simulink model "sampleModel2072_pp_difftest"  (R2021a)
settings: Solver=VariableStepAuto  StartTime=0.0  StopTime=10.0  RelTol=1e-3
undefined symbols (not defined in the file or in its folder): DiscIntNeverNeededParam, magnitude, Newton, Raphson
libraries: simulink x184, pid_lib x33
(part 5 of 5)

== system sampleModel2072_pp_difftest/cfblk57/cfblk10 ==
  cfblk1 : Inport
  cfblk10 : Delay  SampleTime=1
  cfblk11 : Delay  SampleTime=1
  cfblk3 : Delay  ShowEnablePort=on  SampleTime=1
      settings: InputPortMap=u0,e6
  cfblk4 : simulink/Discrete/Difference  ICPrevInput=0.0  OutMin=[]  OutMax=[]  OutDataTypeStr=Inherit: Inherit via back propagation  OutDataType=fixdt(1, 16)  OutScaling=2^-10  DoSatur=off
  cfblk5 : simulink/Discrete/Transfer Fcn Lead or Lag  PoleZ=0.95  ZeroZ=0.75  ICPrevOutput=0.0  ICPrevInput=0.0  DoSatur=off
      settings: SourceProductBaseCode=SL
  cfblk6 : Sqrt  SaturateOnIntegerOverflow=on
  cfblk7 : Product
  cfblk8 : Sum  Inputs=+-
  cfblk9 : Polyval  Coefs=[ +2.081618890e-019, -1.441693666e-014, +4.719686976e-010, -8.536869453e-006, +1.621573104e-001, -8.087801117e+001 ]
  cfblk2 : Outport
  wires:
  cfblk9/1 -> cfblk7/1
  cfblk1/1 -> cfblk4/1
  cfblk5/1 -> cfblk9/1
  cfblk8/1 -> cfblk6/1
  cfblk4/1 -> cfblk3/1, cfblk8/2, cfblk2/1
  cfblk3/1 -> cfblk7/2, cfblk5/1
  cfblk7/1 -> cfblk10/1
  cfblk10/1 -> cfblk3/2
  cfblk6/1 -> cfblk11/1
  cfblk11/1 -> cfblk8/1

== system sampleModel2072_pp_difftest/cfblk57/cfblk11 ==
  cfblk1 : Inport
  cfblk10 : ComplexToRealImag
  cfblk11 : Product
  cfblk12 : simulink/Math Operations/Slider Gain  gain=1  low=0  high=2
  cfblk13 : Squeeze
  cfblk14 : Product  Inputs=*
  cfblk15 : simulink/Math Operations/Slider Gain  gain=1  low=0  high=2
  cfblk16 : Delay  SampleTime=1
  cfblk3 : simulink/Discrete/Difference  ICPrevInput=0.0  OutMin=[]  OutMax=[]  OutDataTypeStr=Inherit: Inherit via back propagation  OutDataType=fixdt(1, 16)  OutScaling=2^-10  DoSatur=off
  cfblk4 : Delay  SampleTime=1
  cfblk5 : pid_lib/PID Controller (2DOF)  Controller=PID  Form=Parallel  TimeDomain=Discrete-time  UseExternalTs=off  SampleTime=1  IntegratorMethod=Forward Euler  FilterMethod=Forward Euler  ControllerParametersSource=internal  P=1  I=1  D=0  UseFilter=on  N=100  b=1  c=1  TunerSelectOption=Transfer Function Based (PID Tuner App)  InitialConditionSource=internal  InitialConditionForIntegrator=0  InitialConditionForFilter=0  DifferentiatorICPrevScaledInput=0  ExternalReset=none  TrackingMode=off  Kt=1  LimitOutput=off  SatLimitsSource=internal  UpperSaturationLimit=inf  LowerSaturationLimit=-inf  LinearizeAsGain=off  AntiWindupMode=none  Kb=1  POutMin=[]  POutMax=[]  IOutMin=[]  IOutMax=[]  DOutMin=[]  DOutMax=[]  NOutMin=[]  NOutMax=[]  bOutMin=[]  bOutMax=[]  cOutMin=[]  cOutMax=[]  SumOutMin=[]  SumOutMax=[]  SaturationOutMin=[]  SaturationOutMax=[]  PParamMin=[]  PParamMax=[]  IParamMin=[]  IParamMax=[]  DParamMin=[]  DParamMax=[]  NParamMin=[]  NParamMax=[]  bParamMin=[]  bParamMax=[]  cParamMin=[]  cParamMax=[]  KbParamMin=[]  KbParamMax=[]  KtParamMin=[]  KtParamMax=[]  KbOutMin=[]  KbOutMax=[]  KtOutMin=[]  KtOutMax=[]  IntegratorOutMin=[]  IntegratorOutMax=[]  FilterOutMin=[]  FilterOutMax=[]  SumI1OutMin=[]  SumI1OutMax=[]  SumI2OutMin=[]  SumI2OutMax=[]  SumI3OutMin=[]  SumI3OutMax=[]  SumI4OutMin=[]  SumI4OutMax=[]  SumDOutMin=[]  SumDOutMax=[]  Sum1OutMin=[]  Sum1OutMax=[]  Sum2OutMin=[]  Sum2OutMax=[]  Sum3OutMin=[]  Sum3OutMax=[]  DifferentiatorOutMin=[]  DifferentiatorOutMax=[]  FilterDiffOutCoefMin=[]  FilterDiffOutCoefMax=[]  ReciprocalOutMin=[]  ReciprocalOutMax=[]  SumDenOutMin=[]  SumDenOutMax=[]  SumNumOutMin=[]  SumNumOutMax=[]  DivideOutMin=[]  DivideOutMax=[]  UdiffTsProdOutMin=[]  UdiffTsProdOutMax=[]  NTsProdOutMin=[]  NTsProdOutMax=[]  UintegralTsProdOutMin=[]  UintegralTsProdOutMax=[]  UngainTsProdOutMin=[]  UngainTsProdOutMax=[]  IntegratorContinuousStateAttributes=''  IntegratorStateMustResolveToSignalObject=off  IntegratorRTWStateStorageClass=Auto  FilterContinuousStateAttributes=''  FilterStateMustResolveToSignalObject=off  FilterRTWStateStorageClass=Auto  ParallelPVariant=InternalParameters  IdealPVariant=Disabled  IVariant=InternalParameters  DVariant=InternalParameters  bVariant=InternalParameters  cVariant=InternalParameters  IntegratorVariant=Discrete  SatVariant=Disabled  AWVariant=Passthrough  PCopyVariant=Disabled  TRVariant=Disabled  FdbkBlocksVariant=Forward  IdealPFdbkVariant=Disabled  SatFdbkVariant=Disabled  DerivativeFilterVariant=ForwardEulerFilter  NVariant=InternalParameters  NCopyVariant=Disabled  FilterICVariant=InternalICsFilter  IntegratorICVariant=InternalICs  ExternalResetVariant=Disabled  TRSumVariant=Passthrough  SumFdbkVariant=Disabled  SumVariant=Sum_PID  TsampFilterVariant=InternalTs  TsampNgainVariant=Passthrough  TsampIntegralVariant=Passthrough  ExternalSaturationOutDataTypeStr=Inherit: Same as second input
      settings: SourceProductBaseCode=SL
  cfblk6 : Sqrt  SaturateOnIntegerOverflow=on
  cfblk7 : PermuteDimensions
  cfblk8 : Sqrt  SaturateOnIntegerOverflow=on
  cfblk9 : Math  Operator=log10  SaturateOnIntegerOverflow=on
  cfblk2 : Outport
  wires:
  cfblk11/1 -> cfblk10/1
  cfblk1/1 -> cfblk14/1
  cfblk3/1 -> cfblk5/1
  cfblk15/1 -> cfblk4/1
  cfblk7/1 -> cfblk8/1, cfblk11/2
  cfblk5/1 -> cfblk2/1
  cfblk12/1 -> cfblk13/1
  cfblk14/1 -> cfblk7/1
  cfblk4/1 -> cfblk9/1
  cfblk10/1 -> cfblk15/1
  cfblk13/1 -> cfblk5/2
  cfblk9/1 -> cfblk12/1
  cfblk6/1 -> cfblk3/1
  cfblk8/1 -> cfblk6/1
  cfblk10/2 -> cfblk16/1
  cfblk16/1 -> cfblk11/1

== system sampleModel2072_pp_difftest/cfblk57/cfblk12 ==
  cfblk1 : Inport
  cfblk10 : simulink/Math Operations/MinMax Running Resettable  Function=min  vinit=0.0
  cfblk11 : Sum  Inputs=+-
  cfblk12 : simulink/Math Operations/Slider Gain  gain=1  low=0  high=2
  cfblk13 : Squeeze
  cfblk14 : Sum
  cfblk3 : DiscreteFilter  SampleTime=1
  cfblk4 : simulink/Discrete/Difference  ICPrevInput=0.0  OutMin=[]  OutMax=[]  OutDataTypeStr=Inherit: Inherit via back propagation  OutDataType=fixdt(1, 16)  OutScaling=2^-10  DoSatur=off
  cfblk5 : pid_lib/PID Controller (2DOF)  Controller=PID  Form=Parallel  TimeDomain=Discrete-time  UseExternalTs=off  SampleTime=1  IntegratorMethod=Forward Euler  FilterMethod=Forward Euler  ControllerParametersSource=internal  P=1  I=1  D=0  UseFilter=on  N=100  b=1  c=1  TunerSelectOption=Transfer Function Based (PID Tuner App)  InitialConditionSource=internal  InitialConditionForIntegrator=0  InitialConditionForFilter=0  DifferentiatorICPrevScaledInput=0  ExternalReset=none  TrackingMode=off  Kt=1  LimitOutput=off  SatLimitsSource=internal  UpperSaturationLimit=inf  LowerSaturationLimit=-inf  LinearizeAsGain=off  AntiWindupMode=none  Kb=1  POutMin=[]  POutMax=[]  IOutMin=[]  IOutMax=[]  DOutMin=[]  DOutMax=[]  NOutMin=[]  NOutMax=[]  bOutMin=[]  bOutMax=[]  cOutMin=[]  cOutMax=[]  SumOutMin=[]  SumOutMax=[]  SaturationOutMin=[]  SaturationOutMax=[]  PParamMin=[]  PParamMax=[]  IParamMin=[]  IParamMax=[]  DParamMin=[]  DParamMax=[]  NParamMin=[]  NParamMax=[]  bParamMin=[]  bParamMax=[]  cParamMin=[]  cParamMax=[]  KbParamMin=[]  KbParamMax=[]  KtParamMin=[]  KtParamMax=[]  KbOutMin=[]  KbOutMax=[]  KtOutMin=[]  KtOutMax=[]  IntegratorOutMin=[]  IntegratorOutMax=[]  FilterOutMin=[]  FilterOutMax=[]  SumI1OutMin=[]  SumI1OutMax=[]  SumI2OutMin=[]  SumI2OutMax=[]  SumI3OutMin=[]  SumI3OutMax=[]  SumI4OutMin=[]  SumI4OutMax=[]  SumDOutMin=[]  SumDOutMax=[]  Sum1OutMin=[]  Sum1OutMax=[]  Sum2OutMin=[]  Sum2OutMax=[]  Sum3OutMin=[]  Sum3OutMax=[]  DifferentiatorOutMin=[]  DifferentiatorOutMax=[]  FilterDiffOutCoefMin=[]  FilterDiffOutCoefMax=[]  ReciprocalOutMin=[]  ReciprocalOutMax=[]  SumDenOutMin=[]  SumDenOutMax=[]  SumNumOutMin=[]  SumNumOutMax=[]  DivideOutMin=[]  DivideOutMax=[]  UdiffTsProdOutMin=[]  UdiffTsProdOutMax=[]  NTsProdOutMin=[]  NTsProdOutMax=[]  UintegralTsProdOutMin=[]  UintegralTsProdOutMax=[]  UngainTsProdOutMin=[]  UngainTsProdOutMax=[]  IntegratorContinuousStateAttributes=''  IntegratorStateMustResolveToSignalObject=off  IntegratorRTWStateStorageClass=Auto  FilterContinuousStateAttributes=''  FilterStateMustResolveToSignalObject=off  FilterRTWStateStorageClass=Auto  ParallelPVariant=InternalParameters  IdealPVariant=Disabled  IVariant=InternalParameters  DVariant=InternalParameters  bVariant=InternalParameters  cVariant=InternalParameters  IntegratorVariant=Discrete  SatVariant=Disabled  AWVariant=Passthrough  PCopyVariant=Disabled  TRVariant=Disabled  FdbkBlocksVariant=Forward  IdealPFdbkVariant=Disabled  SatFdbkVariant=Disabled  DerivativeFilterVariant=ForwardEulerFilter  NVariant=InternalParameters  NCopyVariant=Disabled  FilterICVariant=InternalICsFilter  IntegratorICVariant=InternalICs  ExternalResetVariant=Disabled  TRSumVariant=Passthrough  SumFdbkVariant=Disabled  SumVariant=Sum_PID  TsampFilterVariant=InternalTs  TsampNgainVariant=Passthrough  TsampIntegralVariant=Passthrough  ExternalSaturationOutDataTypeStr=Inherit: Same as second input
      settings: SourceProductBaseCode=SL
  cfblk6 : DiscreteFilter  SampleTime=1
  cfblk7 : ComplexToMagnitudeAngle
  cfblk8 : MinMax  Inputs=2
  cfblk9 : ComplexToMagnitudeAngle
  cfblk2 : Outport
  wires:
  cfblk3/1 -> cfblk11/1
  cfblk13/1 -> cfblk8/1
  cfblk4/1 -> cfblk9/1, cfblk5/1
  cfblk11/1 -> cfblk12/1
  cfblk14/1 -> cfblk2/1
  cfblk10/1 -> cfblk7/1
  cfblk9/1 -> cfblk8/2
  cfblk9/2 -> cfblk10/1, cfblk11/2
  cfblk6/1 -> cfblk4/1
  cfblk1/1 -> cfblk6/1, cfblk5/2
  cfblk5/1 -> cfblk10/2
  cfblk7/1 -> cfblk13/1
  cfblk12/1 -> cfblk14/1
  cfblk7/2 -> cfblk3/1
  cfblk8/1 -> cfblk14/2

== system sampleModel2072_pp_difftest/cfblk58/cfblk10 ==
  cfblk1 : Inport
  cfblk13 : Inport  Port=2
  cfblk10 : Squeeze
  cfblk11 : ComplexToMagnitudeAngle
  cfblk12 : Sum  Inputs=+-
  cfblk15 : Delay  SampleTime=1
  cfblk3 : DiscreteIntegrator  ICPrevOutput=DiscIntNeverNeededParam  ICPrevScaledInput=DiscIntNeverNeededParam
  cfblk4 : DiscreteTransferFcn  SampleTime=1
  cfblk5 : simulink/Discrete/Transfer Fcn Real Zero  ZeroZ=0.75  ICPrevInput=0.0  DoSatur=off
      settings: SourceProductBaseCode=SL
  cfblk6 : DiscreteIntegrator  ICPrevOutput=DiscIntNeverNeededParam  ICPrevScaledInput=DiscIntNeverNeededParam
  cfblk7 : Sum
  cfblk8 : Squeeze
  cfblk9 : Product  Inputs=*
  cfblk2 : Outport
  cfblk14 : Outport  Port=2
  wires:
  cfblk6/1 -> cfblk14/1
  cfblk8/1 -> cfblk11/1
  cfblk1/1 -> cfblk5/1
  cfblk10/1 -> cfblk8/1
  cfblk13/1 -> cfblk9/1
  cfblk3/1 -> cfblk10/1
  cfblk9/1 -> cfblk12/1
  cfblk5/1 -> cfblk2/1
  cfblk12/1 -> cfblk7/1
  cfblk11/1 -> cfblk4/1
  cfblk4/1 -> cfblk12/2, cfblk7/2
  cfblk11/2 -> cfblk6/1
  cfblk7/1 -> cfblk15/1
  cfblk15/1 -> cfblk3/1

== system sampleModel2072_pp_difftest/cfblk58/cfblk11 ==
  cfblk1 : Inport
  cfblk10 : MinMax
  cfblk11 : simulink/Math Operations/Slider Gain  gain=1  low=0  high=2
  cfblk12 : UnaryMinus
  cfblk13 : simulink/Math Operations/MinMax Running Resettable  Function=min  vinit=0.0
  cfblk14 : Trigonometry
  cfblk15 : Sqrt  SaturateOnIntegerOverflow=on
  cfblk16 : Sum  Inputs=|++
  cfblk17 : Delay  SampleTime=1
  cfblk18 : Delay  SampleTime=1
  cfblk3 : DiscreteFir  SampleTime=1
  cfblk4 : simulink/Discrete/Difference  ICPrevInput=0.0  OutMin=[]  OutMax=[]  OutDataTypeStr=Inherit: Inherit via back propagation  OutDataType=fixdt(1, 16)  OutScaling=2^-10  DoSatur=off
  cfblk5 : pid_lib/PID Controller  Controller=PID  Form=Parallel  TimeDomain=Discrete-time  UseExternalTs=off  SampleTime=1  IntegratorMethod=Forward Euler  FilterMethod=Forward Euler  ControllerParametersSource=internal  P=1  I=1  D=0  UseFilter=on  N=100  TunerSelectOption=Transfer Function Based (PID Tuner App)  InitialConditionSource=internal  InitialConditionForIntegrator=0  InitialConditionForFilter=0  DifferentiatorICPrevScaledInput=0  ExternalReset=none  TrackingMode=off  Kt=1  LimitOutput=off  SatLimitsSource=internal  UpperSaturationLimit=inf  LowerSaturationLimit=-inf  LinearizeAsGain=off  AntiWindupMode=none  Kb=1  POutMin=[]  POutMax=[]  IOutMin=[]  IOutMax=[]  DOutMin=[]  DOutMax=[]  NOutMin=[]  NOutMax=[]  SumOutMin=[]  SumOutMax=[]  SaturationOutMin=[]  SaturationOutMax=[]  PParamMin=[]  PParamMax=[]  IParamMin=[]  IParamMax=[]  DParamMin=[]  DParamMax=[]  NParamMin=[]  NParamMax=[]  KbParamMin=[]  KbParamMax=[]  KtParamMin=[]  KtParamMax=[]  KbOutMin=[]  KbOutMax=[]  KtOutMin=[]  KtOutMax=[]  IntegratorOutMin=[]  IntegratorOutMax=[]  FilterOutMin=[]  FilterOutMax=[]  SumI1OutMin=[]  SumI1OutMax=[]  SumI2OutMin=[]  SumI2OutMax=[]  SumI3OutMin=[]  SumI3OutMax=[]  SumI4OutMin=[]  SumI4OutMax=[]  SumDOutMin=[]  SumDOutMax=[]  DifferentiatorOutMin=[]  DifferentiatorOutMax=[]  FilterDiffOutCoefMin=[]  FilterDiffOutCoefMax=[]  ReciprocalOutMin=[]  ReciprocalOutMax=[]  SumDenOutMin=[]  SumDenOutMax=[]  SumNumOutMin=[]  SumNumOutMax=[]  DivideOutMin=[]  DivideOutMax=[]  UdiffTsProdOutMin=[]  UdiffTsProdOutMax=[]  NTsProdOutMin=[]  NTsProdOutMax=[]  UintegralTsProdOutMin=[]  UintegralTsProdOutMax=[]  UngainTsProdOutMin=[]  UngainTsProdOutMax=[]  IntegratorContinuousStateAttributes=''  IntegratorStateMustResolveToSignalObject=off  IntegratorRTWStateStorageClass=Auto  FilterContinuousStateAttributes=''  FilterStateMustResolveToSignalObject=off  FilterRTWStateStorageClass=Auto  ParallelPVariant=InternalParameters  IdealPVariant=Disabled  IVariant=InternalParameters  DVariant=InternalParameters  IntegratorVariant=Discrete  SatVariant=Disabled  AWVariant=Passthrough  PCopyVariant=Disabled  TRVariant=Disabled  FdbkBlocksVariant=Forward  IdealPFdbkVariant=Disabled  SatFdbkVariant=Disabled  DerivativeFilterVariant=ForwardEulerFilter  NVariant=InternalParameters  NCopyVariant=Disabled  FilterICVariant=InternalICsFilter  IntegratorICVariant=InternalICs  ExternalResetVariant=Disabled  TRSumVariant=Passthrough  SumFdbkVariant=Disabled  SumVariant=Sum_PID  TsampFilterVariant=InternalTs  TsampNgainVariant=Passthrough  TsampIntegralVariant=Passthrough  ExternalSaturationOutDataTypeStr=Inherit: Same as second input
  cfblk6 : DiscreteStateSpace
  cfblk7 : Sqrt  SaturateOnIntegerOverflow=on
  cfblk8 : Product
  cfblk9 : simulink/Math Operations/MinMax Running Resettable  Function=min  vinit=0.0
  cfblk2 : Outport
  wires:
  cfblk16/1 -> cfblk13/1, cfblk9/2
  cfblk3/1 -> cfblk7/1
  cfblk12/1 -> cfblk14/1
  cfblk13/1 -> cfblk9/1
  cfblk11/1 -> cfblk2/1
  cfblk7/1 -> cfblk15/1
  cfblk5/1 -> cfblk3/1
  cfblk9/1 -> cfblk8/1, cfblk17/1
  cfblk10/1 -> cfblk6/1, cfblk8/2
  cfblk1/1 -> cfblk5/1
  cfblk8/1 -> cfblk11/1
  cfblk15/1 -> cfblk16/1
  cfblk6/1 -> cfblk12/1
  cfblk4/1 -> cfblk10/1, cfblk16/2
  cfblk17/1 -> cfblk13/2
  cfblk14/1 -> cfblk18/1
  cfblk18/1 -> cfblk4/1

== system sampleModel2072_pp_difftest/cfblk58/cfblk12 ==
  cfblk1 : Inport
  cfblk13 : Inport  Port=2
  cfblk10 : Trigonometry
  cfblk11 : Polyval  Coefs=[ +2.081618890e-019, -1.441693666e-014, +4.719686976e-010, -8.536869453e-006, +1.621573104e-001, -8.087801117e+001 ]
  cfblk12 : Gain  Gain=[407219525.504462]
  cfblk14 : Delay  SampleTime=1
  cfblk3 : DiscreteIntegrator  ICPrevOutput=DiscIntNeverNeededParam  ICPrevScaledInput=DiscIntNeverNeededParam
  cfblk4 : DiscreteZeroPole  Poles=[0 0.5]  Gain=1
  cfblk5 : Delay  ShowEnablePort=on  SampleTime=1
      settings: InputPortMap=u0,e6
  cfblk6 : DiscreteTransferFcn  SampleTime=1
  cfblk7 : Product  Inputs=*
  cfblk8 : Gain  Gain=[-561419441.589536]
  cfblk9 : Signum
  cfblk2 : Outport
  wires:
  cfblk1/1 -> cfblk7/1
  cfblk12/1 -> cfblk6/1
  cfblk3/1 -> cfblk4/1
  cfblk8/1 -> cfblk11/1
  cfblk6/1 -> cfblk5/1
  cfblk9/1 -> cfblk10/1
  cfblk13/1 -> cfblk2/1
  cfblk5/1 -> cfblk8/1
  cfblk10/1 -> cfblk3/1
  cfblk7/1 -> cfblk9/1
  cfblk4/1 -> cfblk12/1
  cfblk11/1 -> cfblk14/1
  cfblk14/1 -> cfblk5/2

== system sampleModel2072_pp_difftest/cfblk58/cfblk7 ==
  cfblk1 : Inport
  cfblk10 : MinMax  Inputs=3
  cfblk11 : Signum
  cfblk12 : ComplexToMagnitudeAngle
  cfblk13 : Product  Inputs=**
  cfblk14 : Polyval  Coefs=[ +2.081618890e-019, -1.441693666e-014, +4.719686976e-010, -8.536869453e-006, +1.621573104e-001, -8.087801117e+001 ]
  cfblk15 : Rounding
  cfblk16 : Assignment  DiagnosticForDimensions=Warning  IndexOptions=Index vector (dialog)  Indices=1  OutputSizes=1
  cfblk17 : Delay  SampleTime=1
  cfblk18 : Delay  SampleTime=1
  cfblk3 : DiscreteFir  SampleTime=1
  cfblk4 : DiscreteFir  SampleTime=1
  cfblk5 : Delay  ShowEnablePort=on  SampleTime=1
      settings: InputPortMap=u0,e6
  cfblk6 : simulink/Math Operations/MinMax Running Resettable  Function=min  vinit=0.0
  cfblk7 : Polyval  Coefs=[ +2.081618890e-019, -1.441693666e-014, +4.719686976e-010, -8.536869453e-006, +1.621573104e-001, -8.087801117e+001 ]
  cfblk8 : Sin  TimeSource=Use external signal  SampleTime=0
  cfblk9 : Abs
  cfblk2 : Outport
  wires:
  cfblk14/1 -> cfblk3/1
  cfblk4/1 -> cfblk15/1
  cfblk13/1 -> cfblk2/1
  cfblk5/1 -> cfblk14/1
  cfblk15/1 -> cfblk16/1
  cfblk8/1 -> cfblk12/1, cfblk5/2
  cfblk6/1 -> cfblk10/1
  cfblk1/1 -> cfblk4/1
  cfblk11/1 -> cfblk13/1
  cfblk16/1 -> cfblk13/2, cfblk7/1
  cfblk7/1 -> cfblk10/2, cfblk10/3
  cfblk3/1 -> cfblk11/1, cfblk9/1
  cfblk12/2 -> cfblk6/1, cfblk6/2
  cfblk10/1 -> cfblk5/1
  cfblk9/1 -> cfblk17/1
  cfblk17/1 -> cfblk16/2
  cfblk12/1 -> cfblk18/1
  cfblk18/1 -> cfblk8/1

== system sampleModel2072_pp_difftest/cfblk58/cfblk8 ==
  cfblk1 : Inport
  cfblk10 : Sin  TimeSource=Use external signal  SampleTime=0
  cfblk11 : Bias  Bias=[681540840.665307]
  cfblk12 : Polyval  Coefs=[ +2.081618890e-019, -1.441693666e-014, +4.719686976e-010, -8.536869453e-006, +1.621573104e-001, -8.087801117e+001 ]
  cfblk13 : ComplexToRealImag
  cfblk14 : PermuteDimensions
  cfblk15 : Abs
  cfblk16 : Sqrt  Operator=rSqrt  AlgorithmType=Newton-Raphson  SaturateOnIntegerOverflow=on
  cfblk17 : Product  Inputs=**
  cfblk18 : Delay  SampleTime=1
  cfblk19 : Delay  SampleTime=1
  cfblk3 : pid_lib/PID Controller (2DOF)  Controller=PID  Form=Parallel  TimeDomain=Discrete-time  UseExternalTs=off  SampleTime=1  IntegratorMethod=Forward Euler  FilterMethod=Forward Euler  ControllerParametersSource=internal  P=1  I=1  D=0  UseFilter=on  N=100  b=1  c=1  TunerSelectOption=Transfer Function Based (PID Tuner App)  InitialConditionSource=internal  InitialConditionForIntegrator=0  InitialConditionForFilter=0  DifferentiatorICPrevScaledInput=0  ExternalReset=none  TrackingMode=off  Kt=1  LimitOutput=off  SatLimitsSource=internal  UpperSaturationLimit=inf  LowerSaturationLimit=-inf  LinearizeAsGain=off  AntiWindupMode=none  Kb=1  POutMin=[]  POutMax=[]  IOutMin=[]  IOutMax=[]  DOutMin=[]  DOutMax=[]  NOutMin=[]  NOutMax=[]  bOutMin=[]  bOutMax=[]  cOutMin=[]  cOutMax=[]  SumOutMin=[]  SumOutMax=[]  SaturationOutMin=[]  SaturationOutMax=[]  PParamMin=[]  PParamMax=[]  IParamMin=[]  IParamMax=[]  DParamMin=[]  DParamMax=[]  NParamMin=[]  NParamMax=[]  bParamMin=[]  bParamMax=[]  cParamMin=[]  cParamMax=[]  KbParamMin=[]  KbParamMax=[]  KtParamMin=[]  KtParamMax=[]  KbOutMin=[]  KbOutMax=[]  KtOutMin=[]  KtOutMax=[]  IntegratorOutMin=[]  IntegratorOutMax=[]  FilterOutMin=[]  FilterOutMax=[]  SumI1OutMin=[]  SumI1OutMax=[]  SumI2OutMin=[]  SumI2OutMax=[]  SumI3OutMin=[]  SumI3OutMax=[]  SumI4OutMin=[]  SumI4OutMax=[]  SumDOutMin=[]  SumDOutMax=[]  Sum1OutMin=[]  Sum1OutMax=[]  Sum2OutMin=[]  Sum2OutMax=[]  Sum3OutMin=[]  Sum3OutMax=[]  DifferentiatorOutMin=[]  DifferentiatorOutMax=[]  FilterDiffOutCoefMin=[]  FilterDiffOutCoefMax=[]  ReciprocalOutMin=[]  ReciprocalOutMax=[]  SumDenOutMin=[]  SumDenOutMax=[]  SumNumOutMin=[]  SumNumOutMax=[]  DivideOutMin=[]  DivideOutMax=[]  UdiffTsProdOutMin=[]  UdiffTsProdOutMax=[]  NTsProdOutMin=[]  NTsProdOutMax=[]  UintegralTsProdOutMin=[]  UintegralTsProdOutMax=[]  UngainTsProdOutMin=[]  UngainTsProdOutMax=[]  IntegratorContinuousStateAttributes=''  IntegratorStateMustResolveToSignalObject=off  IntegratorRTWStateStorageClass=Auto  FilterContinuousStateAttributes=''  FilterStateMustResolveToSignalObject=off  FilterRTWStateStorageClass=Auto  ParallelPVariant=InternalParameters  IdealPVariant=Disabled  IVariant=InternalParameters  DVariant=InternalParameters  bVariant=InternalParameters  cVariant=InternalParameters  IntegratorVariant=Discrete  SatVariant=Disabled  AWVariant=Passthrough  PCopyVariant=Disabled  TRVariant=Disabled  FdbkBlocksVariant=Forward  IdealPFdbkVariant=Disabled  SatFdbkVariant=Disabled  DerivativeFilterVariant=ForwardEulerFilter  NVariant=InternalParameters  NCopyVariant=Disabled  FilterICVariant=InternalICsFilter  IntegratorICVariant=InternalICs  ExternalResetVariant=Disabled  TRSumVariant=Passthrough  SumFdbkVariant=Disabled  SumVariant=Sum_PID  TsampFilterVariant=InternalTs  TsampNgainVariant=Passthrough  TsampIntegralVariant=Passthrough  ExternalSaturationOutDataTypeStr=Inherit: Same as second input
      settings: SourceProductBaseCode=SL
  cfblk4 : simulink/Discrete/Difference  ICPrevInput=0.0  OutMin=[]  OutMax=[]  OutDataTypeStr=Inherit: Inherit via back propagation  OutDataType=fixdt(1, 16)  OutScaling=2^-10  DoSatur=off
  cfblk5 : simulink/Discrete/Tapped Delay  vinit=0.0  samptime=-1  NumDelays=1  DelayOrder=Oldest  includeCurrent=off
  cfblk6 : DiscreteTransferFcn  SampleTime=1
  cfblk7 : DiscreteTransferFcn  SampleTime=1
  cfblk8 : simulink/Discrete/Transfer Fcn First Order  PoleZ=0.95  ICPrevOutput=0.0  DoSatur=off
  cfblk9 : DiscreteTransferFcn  SampleTime=1
  cfblk2 : Outport
  wires:
  cfblk15/1 -> cfblk5/1
  cfblk10/1 -> cfblk11/1
  cfblk3/1 -> cfblk10/1
  cfblk13/1 -> cfblk8/1
  cfblk8/1 -> cfblk12/1
  cfblk13/2 -> cfblk17/2
  cfblk4/1 -> cfblk6/1
  cfblk12/1 -> cfblk3/1
  cfblk1/1 -> cfblk7/1
  cfblk14/1 -> cfblk13/1
  cfblk17/1 -> cfblk9/1
  cfblk6/1 -> cfblk14/1, cfblk15/1
  cfblk7/1 -> cfblk3/2
  cfblk11/1 -> cfblk16/1
  cfblk16/1 -> cfblk2/1
  cfblk9/1 -> cfblk18/1
  cfblk18/1 -> cfblk17/1
  cfblk5/1 -> cfblk19/1
  cfblk19/1 -> cfblk4/1

== system sampleModel2072_pp_difftest/cfblk58/cfblk9 ==
  cfblk1 : Inport
  cfblk10 : Product  Inputs=*
  cfblk11 : Product  Inputs=**
  cfblk12 : UnaryMinus
  cfblk13 : Delay  SampleTime=1
  cfblk14 : Delay  SampleTime=1
  cfblk3 : DiscreteFilter  SampleTime=1
  cfblk4 : simulink/Discrete/Transfer Fcn Real Zero  ZeroZ=0.75  ICPrevInput=0.0  DoSatur=off
      settings: SourceProductBaseCode=SL
  cfblk5 : DiscreteTransferFcn  SampleTime=1
  cfblk6 : DotProduct  InputSameDT=on  OutDataTypeStr=Inherit: Inherit via internal rule
  cfblk7 : Sqrt  Operator=rSqrt  AlgorithmType=Newton-Raphson  SaturateOnIntegerOverflow=on
  cfblk8 : PermuteDimensions
  cfblk9 : Sum  Inputs=|++
  cfblk2 : Outport
  wires:
  cfblk4/1 -> cfblk3/1
  cfblk6/1 -> cfblk8/1
  cfblk8/1 -> cfblk4/1
  cfblk1/1 -> cfblk10/1
  cfblk5/1 -> cfblk12/1
  cfblk10/1 -> cfblk6/2, cfblk7/1
  cfblk11/1 -> cfblk9/1, cfblk2/1
  cfblk7/1 -> cfblk9/2, cfblk11/2
  cfblk3/1 -> cfblk11/1
  cfblk9/1 -> cfblk13/1
  cfblk13/1 -> cfblk6/1
  cfblk12/1 -> cfblk14/1
  cfblk14/1 -> cfblk5/1

== system sampleModel2072_pp_difftest/cfblk59/cfblk12 ==
  cfblk1 : Inport
  cfblk10 : Squeeze
  cfblk11 : Product  Inputs=*
  cfblk12 : Delay  SampleTime=1
  cfblk13 : Delay  SampleTime=1
  cfblk3 : DiscreteTransferFcn  SampleTime=1
  cfblk4 : pid_lib/PID Controller (2DOF)  Controller=PID  Form=Parallel  TimeDomain=Discrete-time  UseExternalTs=off  SampleTime=1  IntegratorMethod=Forward Euler  FilterMethod=Forward Euler  ControllerParametersSource=internal  P=1  I=1  D=0  UseFilter=on  N=100  b=1  c=1  TunerSelectOption=Transfer Function Based (PID Tuner App)  InitialConditionSource=internal  InitialConditionForIntegrator=0  InitialConditionForFilter=0  DifferentiatorICPrevScaledInput=0  ExternalReset=none  TrackingMode=off  Kt=1  LimitOutput=off  SatLimitsSource=internal  UpperSaturationLimit=inf  LowerSaturationLimit=-inf  LinearizeAsGain=off  AntiWindupMode=none  Kb=1  POutMin=[]  POutMax=[]  IOutMin=[]  IOutMax=[]  DOutMin=[]  DOutMax=[]  NOutMin=[]  NOutMax=[]  bOutMin=[]  bOutMax=[]  cOutMin=[]  cOutMax=[]  SumOutMin=[]  SumOutMax=[]  SaturationOutMin=[]  SaturationOutMax=[]  PParamMin=[]  PParamMax=[]  IParamMin=[]  IParamMax=[]  DParamMin=[]  DParamMax=[]  NParamMin=[]  NParamMax=[]  bParamMin=[]  bParamMax=[]  cParamMin=[]  cParamMax=[]  KbParamMin=[]  KbParamMax=[]  KtParamMin=[]  KtParamMax=[]  KbOutMin=[]  KbOutMax=[]  KtOutMin=[]  KtOutMax=[]  IntegratorOutMin=[]  IntegratorOutMax=[]  FilterOutMin=[]  FilterOutMax=[]  SumI1OutMin=[]  SumI1OutMax=[]  SumI2OutMin=[]  SumI2OutMax=[]  SumI3OutMin=[]  SumI3OutMax=[]  SumI4OutMin=[]  SumI4OutMax=[]  SumDOutMin=[]  SumDOutMax=[]  Sum1OutMin=[]  Sum1OutMax=[]  Sum2OutMin=[]  Sum2OutMax=[]  Sum3OutMin=[]  Sum3OutMax=[]  DifferentiatorOutMin=[]  DifferentiatorOutMax=[]  FilterDiffOutCoefMin=[]  FilterDiffOutCoefMax=[]  ReciprocalOutMin=[]  ReciprocalOutMax=[]  SumDenOutMin=[]  SumDenOutMax=[]  SumNumOutMin=[]  SumNumOutMax=[]  DivideOutMin=[]  DivideOutMax=[]  UdiffTsProdOutMin=[]  UdiffTsProdOutMax=[]  NTsProdOutMin=[]  NTsProdOutMax=[]  UintegralTsProdOutMin=[]  UintegralTsProdOutMax=[]  UngainTsProdOutMin=[]  UngainTsProdOutMax=[]  IntegratorContinuousStateAttributes=''  IntegratorStateMustResolveToSignalObject=off  IntegratorRTWStateStorageClass=Auto  FilterContinuousStateAttributes=''  FilterStateMustResolveToSignalObject=off  FilterRTWStateStorageClass=Auto  ParallelPVariant=InternalParameters  IdealPVariant=Disabled  IVariant=InternalParameters  DVariant=InternalParameters  bVariant=InternalParameters  cVariant=InternalParameters  IntegratorVariant=Discrete  SatVariant=Disabled  AWVariant=Passthrough  PCopyVariant=Disabled  TRVariant=Disabled  FdbkBlocksVariant=Forward  IdealPFdbkVariant=Disabled  SatFdbkVariant=Disabled  DerivativeFilterVariant=ForwardEulerFilter  NVariant=InternalParameters  NCopyVariant=Disabled  FilterICVariant=InternalICsFilter  IntegratorICVariant=InternalICs  ExternalResetVariant=Disabled  TRSumVariant=Passthrough  SumFdbkVariant=Disabled  SumVariant=Sum_PID  TsampFilterVariant=InternalTs  TsampNgainVariant=Passthrough  TsampIntegralVariant=Passthrough  ExternalSaturationOutDataTypeStr=Inherit: Same as second input
      settings: SourceProductBaseCode=SL
  cfblk5 : Sum  Inputs=+
  cfblk6 : Gain  Gain=[173048777.474540]
  cfblk7 : Trigonometry
  cfblk8 : MinMax  Inputs=3
  cfblk9 : PermuteDimensions
  cfblk2 : Outport
  wires:
  cfblk5/1 -> cfblk10/1
  cfblk6/1 -> cfblk9/1
  cfblk4/1 -> cfblk7/1
  cfblk7/1 -> cfblk5/1, cfblk12/1
  cfblk8/1 -> cfblk3/1
  cfblk1/1 -> cfblk8/1
  cfblk3/1 -> cfblk11/1
  cfblk9/1 -> cfblk2/1
  cfblk10/1 -> cfblk6/1
  cfblk11/1 -> cfblk4/1, cfblk4/2, cfblk13/1
  cfblk12/1 -> cfblk8/2
  cfblk13/1 -> cfblk8/3

== system sampleModel2072_pp_difftest/cfblk59/cfblk13 ==
  cfblk1 : Inport
  cfblk10 : Sqrt  Operator=rSqrt  AlgorithmType=Newton-Raphson  SaturateOnIntegerOverflow=on
  cfblk11 : Product  Inputs=*
  cfblk12 : DotProduct  InputSameDT=on  OutDataTypeStr=Inherit: Inherit via internal rule
  cfblk13 : Sum  Inputs=--
  cfblk14 : Abs
  cfblk15 : Constant  Value=[-124017775.786354]  SampleTime=1
  cfblk16 : Delay  SampleTime=1
  cfblk17 : Delay  SampleTime=1
  cfblk3 : DiscreteStateSpace
  cfblk4 : Trigonometry
  cfblk5 : ComplexToRealImag
  cfblk6 : simulink/Math Operations/MinMax Running Resettable  Function=min  vinit=0.0
  cfblk7 : Product  Inputs=*
  cfblk8 : Sum  Inputs=+
  cfblk9 : Sqrt  SaturateOnIntegerOverflow=on
  cfblk2 : Outport
  wires:
  cfblk1/1 -> cfblk10/1
  cfblk9/1 -> cfblk14/1
  cfblk7/1 -> cfblk11/1
  cfblk13/1 -> cfblk2/1
  cfblk14/1 -> cfblk4/1, cfblk7/1
  cfblk5/1 -> cfblk8/1
  cfblk6/1 -> cfblk9/1
  cfblk12/1 -> cfblk5/1
  cfblk15/1 -> cfblk3/1
  cfblk5/2 -> cfblk6/2
  cfblk10/1 -> cfblk12/2
  cfblk4/1 -> cfblk13/1
  cfblk3/1 -> cfblk13/2
  cfblk8/1 -> cfblk16/1
  cfblk16/1 -> cfblk12/1
  cfblk11/1 -> cfblk17/1
  cfblk17/1 -> cfblk6/1

== system sampleModel2072_pp_difftest/cfblk60/cfblk6 ==
  cfblk1 : Inport
  cfblk10 : simulink/Math Operations/MinMax Running Resettable  Function=min  vinit=0.0
  cfblk11 : Product  Inputs=*
  cfblk12 : Math  SaturateOnIntegerOverflow=on
  cfblk13 : Product  Inputs=*
  cfblk{14..17} (4 alike) : Delay  SampleTime=1
  cfblk3 : DiscreteTransferFcn  SampleTime=1
  cfblk4 : Product  Inputs=**
  cfblk5 : Trigonometry
  cfblk6 : Rounding
  cfblk7 : Reshape
  cfblk8 : Gain  Gain=[317006020.103301]
  cfblk9 : Sqrt  SaturateOnIntegerOverflow=on
  cfblk2 : Outport
  wires:
  cfblk1/1 -> cfblk2/1
  cfblk8/1 -> cfblk6/1
  cfblk3/1 -> cfblk11/1
  cfblk13/1 -> cfblk12/1
  cfblk7/1 -> cfblk9/1
  cfblk11/1 -> cfblk13/1
  cfblk9/1 -> cfblk10/2, cfblk17/1
  cfblk12/1 -> cfblk4/1
  cfblk4/1 -> cfblk8/1
  cfblk6/1 -> cfblk14/1, cfblk15/1
  cfblk5/1 -> cfblk10/1
  cfblk14/1 -> cfblk4/2
  cfblk15/1 -> cfblk3/1
  cfblk10/1 -> cfblk16/1
  cfblk16/1 -> cfblk5/1
  cfblk17/1 -> cfblk7/1

== system sampleModel2072_pp_difftest/cfblk60/cfblk7 ==
  cfblk1 : Inport
  cfblk3 : Delay  SampleTime=1
  cfblk4 : UnitDelay  HasFrameUpgradeWarning=on
  cfblk5 : simulink/Discrete/Transfer Fcn Real Zero  ZeroZ=0.75  ICPrevInput=0.0  DoSatur=off
      settings: SourceProductBaseCode=SL
  cfblk6 : simulink/Math Operations/MinMax Running Resettable  Function=min  vinit=0.0
  cfblk7 : Assignment  DiagnosticForDimensions=Warning  IndexOptions=Index vector (dialog)  Indices=1  OutputSizes=1
  cfblk8 : Delay  SampleTime=1
  cfblk2 : Outport
  wires:
  cfblk3/1 -> cfblk7/1
  cfblk6/1 -> cfblk2/1
  cfblk1/1 -> cfblk6/1, cfblk3/1
  cfblk4/1 -> cfblk6/2
  cfblk7/1 -> cfblk4/1, cfblk5/1
  cfblk5/1 -> cfblk8/1
  cfblk8/1 -> cfblk7/2

== system sampleModel2072_pp_difftest/cfblk63/cfblk5 ==
  cfblk1 : Inport
  cfblk10 : MinMax  Inputs=3
  cfblk11 : Sum  Inputs=+-
  cfblk12 : ComplexToMagnitudeAngle
  cfblk13 : Product
  cfblk14 : Sum  Inputs=+-
  cfblk15 : MinMax  Function=max  Inputs=2
  cfblk16 : simulink/Math Operations/Slider Gain  gain=1  low=0  high=2
  cfblk17 : Delay
  cfblk3 : simulink/Discrete/Transfer Fcn Lead or Lag  PoleZ=0.95  ZeroZ=0.75  ICPrevOutput=0.0  ICPrevInput=0.0  DoSatur=off
      settings: SourceProductBaseCode=SL
  cfblk4 : Delay  ShowEnablePort=on
      settings: InputPortMap=u0,e6
  cfblk5 : simulink/Discrete/Transfer Fcn First Order  PoleZ=0.95  ICPrevOutput=0.0  DoSatur=off
  cfblk6 : Bias  Bias=[-795958545.295486]
  cfblk7 : Sqrt  Operator=rSqrt  AlgorithmType=Newton-Raphson  SaturateOnIntegerOverflow=on
  cfblk8 : Sqrt  Operator=rSqrt  AlgorithmType=Newton-Raphson  SaturateOnIntegerOverflow=on
  cfblk9 : Sum  Inputs=|++
  cfblk2 : Outport
  wires:
  cfblk14/1 -> cfblk11/1
  cfblk3/1 -> cfblk14/1
  cfblk11/1 -> cfblk5/1, cfblk9/2
  cfblk9/1 -> cfblk13/1
  cfblk1/1 -> cfblk13/2, cfblk16/1
  cfblk15/1 -> cfblk2/1
  cfblk6/1 -> cfblk9/1, cfblk10/3
  cfblk13/1 -> cfblk15/1
  cfblk8/1 -> cfblk7/1
  cfblk7/1 -> cfblk14/2, cfblk4/1
  cfblk16/1 -> cfblk8/1, cfblk3/1
  cfblk12/1 -> cfblk10/1
  cfblk5/1 -> cfblk6/1, cfblk4/2
  cfblk12/2 -> cfblk10/2, cfblk15/2
  cfblk4/1 -> cfblk12/1
  cfblk10/1 -> cfblk17/1
  cfblk17/1 -> cfblk11/2

== system sampleModel2072_pp_difftest/cfblk63/cfblk6 ==
  cfblk1 : Inport
  cfblk15 : Inport  Port=2
  cfblk10 : Assignment  DiagnosticForDimensions=Warning  IndexOptions=Index vector (dialog)  Indices=1  OutputSizes=1
  cfblk11 : Math  Operator=10^u  SaturateOnIntegerOverflow=on
  cfblk12 : Product  Inputs=**
  cfblk13 : PermuteDimensions
  cfblk14 : Math  Operator=square  SaturateOnIntegerOverflow=on
  cfblk16 : Delay
  cfblk17 : Delay
  cfblk18 : Delay
  cfblk3 : DiscreteStateSpace  SampleTime=-1
  cfblk4 : DiscreteTransferFcn
  cfblk5 : DiscreteTransferFcn
  cfblk6 : simulink/Discrete/Tapped Delay  vinit=0.0  samptime=-1  NumDelays=1  DelayOrder=Oldest  includeCurrent=off
  cfblk7 : Product  Inputs=*
  cfblk8 : simulink/Math Operations/Slider Gain  gain=1  low=0  high=2
  cfblk9 : Assignment  DiagnosticForDimensions=Warning  IndexOptions=Index vector (dialog)  Indices=1  OutputSizes=1
  cfblk2 : Outport
  wires:
  cfblk14/1 -> cfblk6/1
  cfblk11/1 -> cfblk10/1
  cfblk7/1 -> cfblk11/1, cfblk9/2
  cfblk13/1 -> cfblk14/1
  cfblk3/1 -> cfblk12/1
  cfblk1/1 -> cfblk5/1
  cfblk12/1 -> cfblk8/1
  cfblk15/1 -> cfblk10/2
  cfblk5/1 -> cfblk2/1, cfblk3/1
  cfblk4/1 -> cfblk13/1
  cfblk8/1 -> cfblk9/1
  cfblk9/1 -> cfblk16/1
  cfblk16/1 -> cfblk12/2
  cfblk6/1 -> cfblk17/1
  cfblk17/1 -> cfblk4/1
  cfblk10/1 -> cfblk18/1
  cfblk18/1 -> cfblk7/1

== system sampleModel2072_pp_difftest/cfblk63/cfblk7 ==
  cfblk1 : Inport
  cfblk10 : Assignment  DiagnosticForDimensions=Warning  IndexOptions=Index vector (dialog)  Indices=1  OutputSizes=1
  cfblk11 : Product
  cfblk12 : Delay
  cfblk13 : Delay
  cfblk14 : Delay
  cfblk3 : simulink/Discrete/Tapped Delay  vinit=0.0  samptime=-1  NumDelays=1  DelayOrder=Oldest  includeCurrent=off
  cfblk4 : UnitDelay  SampleTime=-1  HasFrameUpgradeWarning=on
  cfblk5 : simulink/Discrete/Tapped Delay  vinit=0.0  samptime=-1  NumDelays=1  DelayOrder=Oldest  includeCurrent=off
  cfblk6 : Product
  cfblk7 : Sum  Inputs=|++
  cfblk8 : DotProduct  InputSameDT=on  OutDataTypeStr=Inherit: Inherit via internal rule
  cfblk9 : Polyval  Coefs=[ +2.081618890e-019, -1.441693666e-014, +4.719686976e-010, -8.536869453e-006, +1.621573104e-001, -8.087801117e+001 ]
  cfblk2 : Outport
  wires:
  cfblk4/1 -> cfblk10/1, cfblk7/2, cfblk10/2, cfblk8/2
  cfblk3/1 -> cfblk4/1
  cfblk6/1 -> cfblk11/1
  cfblk5/1 -> cfblk8/1, cfblk13/1
  cfblk11/1 -> cfblk3/1
  cfblk1/1 -> cfblk6/1
  cfblk7/1 -> cfblk5/1
  cfblk8/1 -> cfblk9/1
  cfblk10/1 -> cfblk2/1, cfblk12/1
  cfblk12/1 -> cfblk11/2
  cfblk13/1 -> cfblk7/1
  cfblk9/1 -> cfblk14/1
  cfblk14/1 -> cfblk6/2

== system sampleModel2072_pp_difftest/cfblk64/cfblk6 ==
  cfblk1 : Inport
  cfblk10 : ComplexToMagnitudeAngle
  cfblk11 : Sum  Inputs=+
  cfblk12 : Gain  Gain=[438041377.944004]
  cfblk13 : Polyval  Coefs=[ +2.081618890e-019, -1.441693666e-014, +4.719686976e-010, -8.536869453e-006, +1.621573104e-001, -8.087801117e+001 ]
  cfblk14 : Delay
  cfblk15 : Delay
  cfblk3 : Delay  ShowEnablePort=on
      settings: InputPortMap=u0,e6
  cfblk4 : Delay  DelayLengthSource=Input port
      settings: InputPortMap=u0,p1
  cfblk5 : DiscreteTransferFcn
  cfblk6 : Sum
  cfblk7 : Assignment  DiagnosticForDimensions=Warning  IndexOptions=Index vector (dialog)  Indices=1  OutputSizes=1
  cfblk8 : Sum  Inputs=+
  cfblk9 : ComplexToMagnitudeAngle
  cfblk2 : Outport
  wires:
  cfblk10/1 -> cfblk6/1
  cfblk10/2 -> cfblk13/1, cfblk7/2
  cfblk6/1 -> cfblk12/1
  cfblk11/1 -> cfblk9/1
  cfblk12/1 -> cfblk4/2, cfblk14/1
  cfblk7/1 -> cfblk5/1
  cfblk13/1 -> cfblk4/1
  cfblk9/1 -> cfblk2/1
  cfblk8/1 -> cfblk11/1
  cfblk4/1 -> cfblk8/1
  cfblk3/1 -> cfblk10/1
  cfblk1/1 -> cfblk3/2
  cfblk9/2 -> cfblk7/1
  cfblk14/1 -> cfblk6/2
  cfblk5/1 -> cfblk15/1
  cfblk15/1 -> cfblk3/1

== system sampleModel2072_pp_difftest/cfblk64/cfblk7 ==
  cfblk1 : Inport
  cfblk10 : Trigonometry
  cfblk11 : DotProduct  InputSameDT=on  OutDataTypeStr=Inherit: Inherit via internal rule
  cfblk12 : Sqrt  SaturateOnIntegerOverflow=on
  cfblk13 : ComplexToMagnitudeAngle
  cfblk14 : MinMax  Inputs=3
  cfblk15 : Delay
  cfblk3 : Delay  DelayLengthSource=Input port
      settings: InputPortMap=u0,p1
  cfblk4 : simulink/Discrete/Transfer Fcn First Order  PoleZ=0.95  ICPrevOutput=0.0  DoSatur=off
  cfblk5 : Reshape
  cfblk6 : Abs
  cfblk7 : Trigonometry
  cfblk8 : Product
  cfblk9 : Sqrt  SaturateOnIntegerOverflow=on
  cfblk2 : Outport
  wires:
  cfblk4/1 -> cfblk6/1
  cfblk13/1 -> cfblk14/1
  cfblk14/1 -> cfblk3/1
  cfblk7/1 -> cfblk9/1
  cfblk6/1 -> cfblk11/2
  cfblk8/1 -> cfblk12/1
  cfblk13/2 -> cfblk2/1
  cfblk9/1 -> cfblk4/1
  cfblk1/1 -> cfblk7/1, cfblk5/1, cfblk8/2
  cfblk5/1 -> cfblk10/1, cfblk14/3
  cfblk10/1 -> cfblk3/2
  cfblk11/1 -> cfblk13/1, cfblk8/1
  cfblk12/1 -> cfblk14/2
  cfblk3/1 -> cfblk15/1
  cfblk15/1 -> cfblk11/1

== system sampleModel2072_pp_difftest/cfblk65/cfblk8 ==
  cfblk1 : Inport
  cfblk10 : Delay
  cfblk3 : simulink/Discrete/Transfer Fcn Real Zero  ZeroZ=0.75  ICPrevInput=0.0  DoSatur=off
      settings: SourceProductBaseCode=SL
  cfblk4 : Assignment  DiagnosticForDimensions=Warning  IndexOptions=Index vector (dialog)  Indices=1  OutputSizes=1
  cfblk5 : Trigonometry
  cfblk6 : Polyval  Coefs=[ +2.081618890e-019, -1.441693666e-014, +4.719686976e-010, -8.536869453e-006, +1.621573104e-001, -8.087801117e+001 ]
  cfblk7 : Bias  Bias=[-920227344.841567]
  cfblk8 : UnaryMinus
  cfblk9 : Delay
  cfblk2 : Outport
  wires:
  cfblk1/1 -> cfblk6/1
  cfblk7/1 -> cfblk4/2, cfblk10/1
  cfblk3/1 -> cfblk4/1
  cfblk8/1 -> cfblk7/1
  cfblk6/1 -> cfblk2/1
  cfblk5/1 -> cfblk8/1
  cfblk4/1 -> cfblk9/1
  cfblk9/1 -> cfblk3/1
  cfblk10/1 -> cfblk5/1

== system sampleModel2072_pp_difftest/cfblk66/cfblk10 ==
  cfblk1 : Inport
  cfblk10 : simulink/Math Operations/MinMax Running Resettable  Function=min  vinit=0.0
  cfblk11 : Product
  cfblk12 : Math  Operator=mod  SaturateOnIntegerOverflow=on
  cfblk13 : Sin  TimeSource=Use external signal  SampleTime=0
  cfblk15 : Delay
  cfblk16 : Delay
  cfblk3 : DiscreteStateSpace  SampleTime=-1
  cfblk4 : simulink/Discrete/Transfer Fcn Lead or Lag  PoleZ=0.95  ZeroZ=0.75  ICPrevOutput=0.0  ICPrevInput=0.0  DoSatur=off
      settings: SourceProductBaseCode=SL
  cfblk5 : DiscreteIntegrator  SampleTime=-1  ICPrevOutput=DiscIntNeverNeededParam  ICPrevScaledInput=DiscIntNeverNeededParam
  cfblk6 : Squeeze
  cfblk7 : Assignment  DiagnosticForDimensions=Warning  IndexOptions=Index vector (dialog)  Indices=1  OutputSizes=1
  cfblk8 : Polyval  Coefs=[ +2.081618890e-019, -1.441693666e-014, +4.719686976e-010, -8.536869453e-006, +1.621573104e-001, -8.087801117e+001 ]
  cfblk9 : Math  Operator=pow  SaturateOnIntegerOverflow=on
  cfblk2 : Outport
  cfblk14 : Outport  Port=2
  wires:
  cfblk8/1 -> cfblk10/2, cfblk16/1
  cfblk7/1 -> cfblk6/1
  cfblk6/1 -> cfblk11/1
  cfblk12/1 -> cfblk10/1
  cfblk5/1 -> cfblk2/1, cfblk7/2
  cfblk10/1 -> cfblk3/1, cfblk9/2, cfblk5/1
  cfblk9/1 -> cfblk7/1
  cfblk11/1 -> cfblk14/1
  cfblk13/1 -> cfblk8/1
  cfblk4/1 -> cfblk13/1, cfblk9/1
  cfblk1/1 -> cfblk12/1
  cfblk3/1 -> cfblk11/2, cfblk15/1
  cfblk15/1 -> cfblk12/2
  cfblk16/1 -> cfblk4/1

== system sampleModel2072_pp_difftest/cfblk66/cfblk11 ==
  cfblk1 : Inport
  cfblk10 : Sum  Inputs=+-
  cfblk11 : simulink/Math Operations/Slider Gain  gain=1  low=0  high=2
  cfblk12 : simulink/Math Operations/Slider Gain  gain=1  low=0  high=2
  cfblk13 : Product  Inputs=**
  cfblk3 : simulink/Discrete/Tapped Delay  vinit=0.0  samptime=-1  NumDelays=1  DelayOrder=Oldest  includeCurrent=off
  cfblk4 : DiscreteFilter
  cfblk5 : DiscreteFir
  cfblk6 : simulink/Discrete/Difference  ICPrevInput=0.0  OutMin=[]  OutMax=[]  OutDataTypeStr=Inherit: Inherit via back propagation  OutDataType=fixdt(1, 16)  OutScaling=2^-10  DoSatur=off
  cfblk7 : Product  Inputs=*
  cfblk8 : Product  Inputs=*
  cfblk9 : Trigonometry
  cfblk2 : Outport
  wires:
  cfblk13/1 -> cfblk7/1
  cfblk12/1 -> cfblk11/1, cfblk10/2
  cfblk9/1 -> cfblk4/1
  cfblk7/1 -> cfblk2/1
  cfblk6/1 -> cfblk13/1
  cfblk8/1 -> cfblk12/1
  cfblk10/1 -> cfblk13/2
  cfblk1/1 -> cfblk8/1
  cfblk4/1 -> cfblk3/1, cfblk10/1
  cfblk5/1 -> cfblk9/1
  cfblk3/1 -> cfblk6/1
  cfblk11/1 -> cfblk5/1

== system sampleModel2072_pp_difftest/cfblk66/cfblk14 ==
  cfblk1 : Inport
  Action Port : ActionPort  ActionPortLabel=if(u1 >= 0)
  cfblk10 : Abs
  cfblk11 : Delay
  cfblk12 : Delay
  cfblk3 : simulink/Discrete/Transfer Fcn Lead or Lag  PoleZ=0.95  ZeroZ=0.75  ICPrevOutput=0.0  ICPrevInput=0.0  DoSatur=off
      settings: SourceProductBaseCode=SL
  cfblk4 : simulink/Discrete/Transfer Fcn Real Zero  ZeroZ=0.75  ICPrevInput=0.0  DoSatur=off
      settings: SourceProductBaseCode=SL
  cfblk5 : UnaryMinus
  cfblk6 : Abs
  cfblk7 : Sqrt  SaturateOnIntegerOverflow=on
  cfblk8 : Sqrt  SaturateOnIntegerOverflow=on
  cfblk9 : Product  Inputs=**
  cfblk2 : Outport
  wires:
  cfblk10/1 -> cfblk7/1, cfblk11/1
  cfblk5/1 -> cfblk6/1
  cfblk3/1 -> cfblk8/1
  cfblk1/1 -> cfblk9/1
  cfblk7/1 -> cfblk4/1
  cfblk4/1 -> cfblk2/1
  cfblk8/1 -> cfblk10/1
  cfblk9/1 -> cfblk3/1
  cfblk11/1 -> cfblk9/2
  cfblk6/1 -> cfblk12/1
  cfblk12/1 -> cfblk5/1

== system sampleModel2072_pp_difftest/cfblk66/cfblk15 ==
  cfblk1 : Inport
  Action Port : ActionPort  ActionPortLabel=else
  cfblk10 : simulink/Math Operations/Slider Gain  gain=1  low=0  high=2
  cfblk11 : Product
  cfblk12 : Sum  Inputs=+
  cfblk13 : Product  Inputs=**
  cfblk14 : Sin  TimeSource=Use external signal  SampleTime=0
  cfblk15 : UnaryMinus
  cfblk16 : Delay
  cfblk17 : Delay
  cfblk3 : pid_lib/PID Controller (2DOF)  Controller=PID  Form=Parallel  TimeDomain=Discrete-time  UseExternalTs=off  SampleTime=-1  IntegratorMethod=Forward Euler  FilterMethod=Forward Euler  ControllerParametersSource=internal  P=1  I=1  D=0  UseFilter=on  N=100  b=1  c=1  TunerSelectOption=Transfer Function Based (PID Tuner App)  InitialConditionSource=internal  InitialConditionForIntegrator=0  InitialConditionForFilter=0  DifferentiatorICPrevScaledInput=0  ExternalReset=none  TrackingMode=off  Kt=1  LimitOutput=off  SatLimitsSource=internal  UpperSaturationLimit=inf  LowerSaturationLimit=-inf  LinearizeAsGain=off  AntiWindupMode=none  Kb=1  POutMin=[]  POutMax=[]  IOutMin=[]  IOutMax=[]  DOutMin=[]  DOutMax=[]  NOutMin=[]  NOutMax=[]  bOutMin=[]  bOutMax=[]  cOutMin=[]  cOutMax=[]  SumOutMin=[]  SumOutMax=[]  SaturationOutMin=[]  SaturationOutMax=[]  PParamMin=[]  PParamMax=[]  IParamMin=[]  IParamMax=[]  DParamMin=[]  DParamMax=[]  NParamMin=[]  NParamMax=[]  bParamMin=[]  bParamMax=[]  cParamMin=[]  cParamMax=[]  KbParamMin=[]  KbParamMax=[]  KtParamMin=[]  KtParamMax=[]  KbOutMin=[]  KbOutMax=[]  KtOutMin=[]  KtOutMax=[]  IntegratorOutMin=[]  IntegratorOutMax=[]  FilterOutMin=[]  FilterOutMax=[]  SumI1OutMin=[]  SumI1OutMax=[]  SumI2OutMin=[]  SumI2OutMax=[]  SumI3OutMin=[]  SumI3OutMax=[]  SumI4OutMin=[]  SumI4OutMax=[]  SumDOutMin=[]  SumDOutMax=[]  Sum1OutMin=[]  Sum1OutMax=[]  Sum2OutMin=[]  Sum2OutMax=[]  Sum3OutMin=[]  Sum3OutMax=[]  DifferentiatorOutMin=[]  DifferentiatorOutMax=[]  FilterDiffOutCoefMin=[]  FilterDiffOutCoefMax=[]  ReciprocalOutMin=[]  ReciprocalOutMax=[]  SumDenOutMin=[]  SumDenOutMax=[]  SumNumOutMin=[]  SumNumOutMax=[]  DivideOutMin=[]  DivideOutMax=[]  UdiffTsProdOutMin=[]  UdiffTsProdOutMax=[]  NTsProdOutMin=[]  NTsProdOutMax=[]  UintegralTsProdOutMin=[]  UintegralTsProdOutMax=[]  UngainTsProdOutMin=[]  UngainTsProdOutMax=[]  IntegratorContinuousStateAttributes=''  IntegratorStateMustResolveToSignalObject=off  IntegratorRTWStateStorageClass=Auto  FilterContinuousStateAttributes=''  FilterStateMustResolveToSignalObject=off  FilterRTWStateStorageClass=Auto  ParallelPVariant=InternalParameters  IdealPVariant=Disabled  IVariant=InternalParameters  DVariant=InternalParameters  bVariant=InternalParameters  cVariant=InternalParameters  IntegratorVariant=Discrete  SatVariant=Disabled  AWVariant=Passthrough  PCopyVariant=Disabled  TRVariant=Disabled  FdbkBlocksVariant=Forward  IdealPFdbkVariant=Disabled  SatFdbkVariant=Disabled  DerivativeFilterVariant=ForwardEulerFilter  NVariant=InternalParameters  NCopyVariant=Disabled  FilterICVariant=InternalICsFilter  IntegratorICVariant=InternalICs  ExternalResetVariant=Disabled  TRSumVariant=Passthrough  SumFdbkVariant=Disabled  SumVariant=Sum_PID  TsampFilterVariant=InternalTs  TsampNgainVariant=Passthrough  TsampIntegralVariant=Passthrough  ExternalSaturationOutDataTypeStr=Inherit: Same as second input
      settings: SourceProductBaseCode=SL
  cfblk4 : DiscreteFilter
  cfblk5 : DiscreteFilter
  cfblk6 : simulink/Discrete/Transfer Fcn Real Zero  ZeroZ=0.75  ICPrevInput=0.0  DoSatur=off
      settings: SourceProductBaseCode=SL
  cfblk7 : simulink/Math Operations/MinMax Running Resettable  Function=min  vinit=0.0
  cfblk8 : Sum  Inputs=+-
  cfblk9 : Product  Inputs=**
  cfblk2 : Outport
  wires:
  cfblk13/1 -> cfblk2/1
  cfblk15/1 -> cfblk13/1
  cfblk14/1 -> cfblk6/1, cfblk12/1
  cfblk7/1 -> cfblk14/1
  cfblk9/1 -> cfblk5/1
  cfblk4/1 -> cfblk10/1, cfblk7/2, cfblk8/2, cfblk13/2
  cfblk10/1 -> cfblk11/1, cfblk9/2
  cfblk1/1 -> cfblk11/2
  cfblk11/1 -> cfblk3/1
  cfblk8/1 -> cfblk7/1
  cfblk3/1 -> cfblk15/1
  cfblk6/1 -> cfblk3/2
  cfblk5/1 -> cfblk8/1, cfblk16/1
  cfblk16/1 -> cfblk9/1
  cfblk12/1 -> cfblk17/1
  cfblk17/1 -> cfblk4/1

== system sampleModel2072_pp_difftest/cfblk66/cfblk9 ==
  cfblk1 : Inport
  cfblk10 : Sqrt  SaturateOnIntegerOverflow=on
  cfblk11 : Sum  Inputs=+
  cfblk12 : PermuteDimensions
  cfblk13 : MinMax  Inputs=2
  cfblk14 : Assignment  DiagnosticForDimensions=Warning  IndexOptions=Index vector (dialog)  Indices=1  OutputSizes=1
  cfblk15 : ComplexToMagnitudeAngle
  cfblk16 : Product
  cfblk17 : Delay
  cfblk18 : Delay
  cfblk3 : simulink/Discrete/Tapped Delay  vinit=0.0  samptime=-1  NumDelays=1  DelayOrder=Oldest  includeCurrent=off
  cfblk4 : DiscreteIntegrator  SampleTime=-1  ICPrevOutput=DiscIntNeverNeededParam  ICPrevScaledInput=DiscIntNeverNeededParam
  cfblk5 : DotProduct  InputSameDT=on  OutDataTypeStr=Inherit: Inherit via internal rule
  cfblk6 : Abs
  cfblk7 : DotProduct  InputSameDT=on  OutDataTypeStr=Inherit: Inherit via internal rule
  cfblk8 : Trigonometry
  cfblk9 : Math  Operator=magnitude^2  SaturateOnIntegerOverflow=on
  cfblk2 : Outport
  wires:
  cfblk11/1 -> cfblk3/1
  cfblk1/1 -> cfblk2/1, cfblk4/1
  cfblk7/1 -> cfblk6/1
  cfblk10/1 -> cfblk16/2
  cfblk9/1 -> cfblk13/1, cfblk11/1
  cfblk15/1 -> cfblk5/1
  cfblk3/1 -> cfblk13/2
  cfblk12/1 -> cfblk15/1
  cfblk14/1 -> cfblk10/1, cfblk7/2
  cfblk4/1 -> cfblk14/2
  cfblk8/1 -> cfblk7/1
  cfblk15/2 -> cfblk8/1
  cfblk16/1 -> cfblk12/1, cfblk9/1
  cfblk13/1 -> cfblk5/2
  cfblk5/1 -> cfblk17/1
  cfblk17/1 -> cfblk16/1
  cfblk6/1 -> cfblk18/1
  cfblk18/1 -> cfblk14/1
